simulink model "quadcopter_sim"  (R2023b)
settings: Solver=ode3  StartTime=0  StopTime=20  FixedStep=0.005  RelTol=1e-3  EnableMultiTasking=on
values from neighbouring files (symbols this model uses):
  g = 9.82    [quadcopter_par.m]
  Ic_x = inertia_matrix(m_x, p_x)    [quadcopter_par.m]
  M_RB = [ mass*eye(3) , zeros(3) ; zeros(3) , Ic_x ]    [quadcopter_par.m]
  mass = sum(m_x)    [quadcopter_par.m]
libraries: aerolibutil x14, sharedtransform x13, slpidlib x6, sharedutil x6, simulink_extras x5, matrix_library x5, vrlib x2, shareduavrstlib x1
(part 2 of 2)

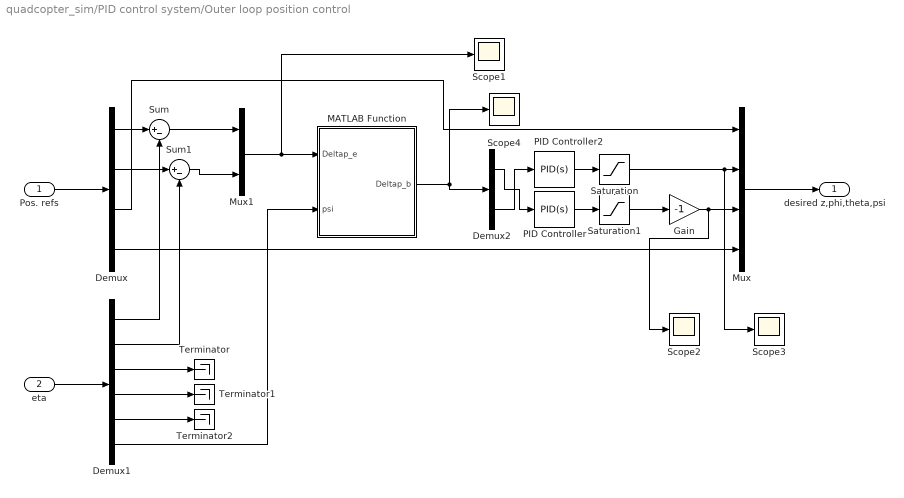
== system quadcopter_sim/PID control system/Outer loop position control ==
  Pos. refs : Inport
  eta : Inport  Port=2
  Demux : Demux
  Demux1 : Demux  Outputs=6
  Demux2 : Demux  Outputs=2
  Gain : Gain  Gain=-1
  MATLAB Function : MATLAB Function  TreatAsAtomicUnit=on
  Mux : Mux
  Mux1 : Mux  Inputs=2
  PID Controller : slpidlib/PID Controller  Controller=PID  Form=Parallel  TimeDomain=Continuous-time  UseExternalTs=off  SampleTime=-1  IntegratorMethod=Forward Euler  FilterMethod=Forward Euler  ControllerParametersSource=internal  P=10  I=0  UseKiTs=off  D=20  N=100  UseFilter=on  TunerSelectOption=Transfer Function Based (PID Tuner App)  InitialConditionSource=internal  InitialConditionForIntegrator=0  InitialConditionForFilter=0  DifferentiatorICPrevScaledInput=0  ExternalReset=none  TrackingMode=off  Kt=1  LimitOutput=off  SatLimitsSource=internal  UpperSaturationLimit=100  LowerSaturationLimit=-100  LinearizeAsGain=on  AntiWindupMode=none  Kb=1  LimitIntegrator=off  UpperIntegratorSaturationLimit=inf  LowerIntegratorSaturationLimit=-inf  POutMin=[]  POutMax=[]  IOutMin=[]  IOutMax=[]  DOutMin=[]  DOutMax=[]  NOutMin=[]  NOutMax=[]  SumOutMin=[]  SumOutMax=[]  SaturationOutMin=[]  SaturationOutMax=[]  PParamMin=[]  PParamMax=[]  IParamMin=[]  IParamMax=[]  DParamMin=[]  DParamMax=[]  NParamMin=[]  NParamMax=[]  KbParamMin=[]  KbParamMax=[]  KtParamMin=[]  KtParamMax=[]  KbOutMin=[]  KbOutMax=[]  KtOutMin=[]  KtOutMax=[]  IntegratorOutMin=[]  IntegratorOutMax=[]  FilterOutMin=[]  FilterOutMax=[]  SumI1OutMin=[]  SumI1OutMax=[]  SumI2OutMin=[]  SumI2OutMax=[]  SumI3OutMin=[]  SumI3OutMax=[]  SumI4OutMin=[]  SumI4OutMax=[]  SumDOutMin=[]  SumDOutMax=[]  DifferentiatorOutMin=[]  DifferentiatorOutMax=[]  FilterDiffOutCoefMin=[]  FilterDiffOutCoefMax=[]  ReciprocalOutMin=[]  ReciprocalOutMax=[]  SumDenOutMin=[]  SumDenOutMax=[]  SumNumOutMin=[]  SumNumOutMax=[]  DivideOutMin=[]  DivideOutMax=[]  UdiffTsProdOutMin=[]  UdiffTsProdOutMax=[]  NTsProdOutMin=[]  NTsProdOutMax=[]  UintegralTsProdOutMin=[]  UintegralTsProdOutMax=[]  UngainTsProdOutMin=[]  UngainTsProdOutMax=[]  ClampingZeroOutDataTypeStr=Inherit: Inherit via back propagation  ClampingZeroOutMin=[]  ClampingZeroOutMax=[]  FilterDenConstantOutDataTypeStr=Inherit: Inherit via back propagation  FilterDenConstantOutMin=[]  FilterDenConstantOutMax=[]  PCopyOutDataTypeStr=Inherit: Inherit via back propagation  PCopyOutMin=[]  PCopyOutMax=[]  NCopyOutDataTypeStr=Inherit: Inherit via back propagation  NCopyOutMin=[]  NCopyOutMax=[]  IntegratorContinuousStateAttributes=''  IntegratorStateMustResolveToSignalObject=off  IntegratorRTWStateStorageClass=Auto  FilterContinuousStateAttributes=''  FilterStateMustResolveToSignalObject=off  FilterRTWStateStorageClass=Auto  ParallelPVariant=InternalParameters  IdealPVariant=Disabled  IVariant=InternalParameters  DVariant=InternalParameters  IntegratorVariant=Continuous  SatVariant=Disabled  AWVariant=Passthrough  PCopyVariant=Disabled  TRVariant=Disabled  FdbkBlocksVariant=Forward  IdealPFdbkVariant=Disabled  SatFdbkVariant=Disabled  DerivativeFilterVariant=ContFilter  NVariant=InternalParameters  NCopyVariant=Disabled  FilterICVariant=InternalICsFilter  IntegratorICVariant=InternalICs  ExternalResetVariant=Disabled  TRSumVariant=Passthrough  SumFdbkVariant=Disabled  SumVariant=Sum_PID  TsampFilterVariant=InternalTs  TsampNgainVariant=Passthrough  TsampIntegralVariant=Disabled_SignalSpec  ExternalSaturationOutDataTypeStr=Inherit: Same as second input
  PID Controller2 : slpidlib/PID Controller  Controller=PID  Form=Parallel  TimeDomain=Continuous-time  UseExternalTs=off  SampleTime=-1  IntegratorMethod=Forward Euler  FilterMethod=Forward Euler  ControllerParametersSource=internal  P=10  I=0  UseKiTs=off  D=20  N=100  UseFilter=on  TunerSelectOption=Transfer Function Based (PID Tuner App)  InitialConditionSource=internal  InitialConditionForIntegrator=0  InitialConditionForFilter=0  DifferentiatorICPrevScaledInput=0  ExternalReset=none  TrackingMode=off  Kt=1  LimitOutput=off  SatLimitsSource=internal  UpperSaturationLimit=100  LowerSaturationLimit=-100  LinearizeAsGain=on  AntiWindupMode=none  Kb=1  LimitIntegrator=off  UpperIntegratorSaturationLimit=inf  LowerIntegratorSaturationLimit=-inf  POutMin=[]  POutMax=[]  IOutMin=[]  IOutMax=[]  DOutMin=[]  DOutMax=[]  NOutMin=[]  NOutMax=[]  SumOutMin=[]  SumOutMax=[]  SaturationOutMin=[]  SaturationOutMax=[]  PParamMin=[]  PParamMax=[]  IParamMin=[]  IParamMax=[]  DParamMin=[]  DParamMax=[]  NParamMin=[]  NParamMax=[]  KbParamMin=[]  KbParamMax=[]  KtParamMin=[]  KtParamMax=[]  KbOutMin=[]  KbOutMax=[]  KtOutMin=[]  KtOutMax=[]  IntegratorOutMin=[]  IntegratorOutMax=[]  FilterOutMin=[]  FilterOutMax=[]  SumI1OutMin=[]  SumI1OutMax=[]  SumI2OutMin=[]  SumI2OutMax=[]  SumI3OutMin=[]  SumI3OutMax=[]  SumI4OutMin=[]  SumI4OutMax=[]  SumDOutMin=[]  SumDOutMax=[]  DifferentiatorOutMin=[]  DifferentiatorOutMax=[]  FilterDiffOutCoefMin=[]  FilterDiffOutCoefMax=[]  ReciprocalOutMin=[]  ReciprocalOutMax=[]  SumDenOutMin=[]  SumDenOutMax=[]  SumNumOutMin=[]  SumNumOutMax=[]  DivideOutMin=[]  DivideOutMax=[]  UdiffTsProdOutMin=[]  UdiffTsProdOutMax=[]  NTsProdOutMin=[]  NTsProdOutMax=[]  UintegralTsProdOutMin=[]  UintegralTsProdOutMax=[]  UngainTsProdOutMin=[]  UngainTsProdOutMax=[]  ClampingZeroOutDataTypeStr=Inherit: Inherit via back propagation  ClampingZeroOutMin=[]  ClampingZeroOutMax=[]  FilterDenConstantOutDataTypeStr=Inherit: Inherit via back propagation  FilterDenConstantOutMin=[]  FilterDenConstantOutMax=[]  PCopyOutDataTypeStr=Inherit: Inherit via back propagation  PCopyOutMin=[]  PCopyOutMax=[]  NCopyOutDataTypeStr=Inherit: Inherit via back propagation  NCopyOutMin=[]  NCopyOutMax=[]  IntegratorContinuousStateAttributes=''  IntegratorStateMustResolveToSignalObject=off  IntegratorRTWStateStorageClass=Auto  FilterContinuousStateAttributes=''  FilterStateMustResolveToSignalObject=off  FilterRTWStateStorageClass=Auto  ParallelPVariant=InternalParameters  IdealPVariant=Disabled  IVariant=InternalParameters  DVariant=InternalParameters  IntegratorVariant=Continuous  SatVariant=Disabled  AWVariant=Passthrough  PCopyVariant=Disabled  TRVariant=Disabled  FdbkBlocksVariant=Forward  IdealPFdbkVariant=Disabled  SatFdbkVariant=Disabled  DerivativeFilterVariant=ContFilter  NVariant=InternalParameters  NCopyVariant=Disabled  FilterICVariant=InternalICsFilter  IntegratorICVariant=InternalICs  ExternalResetVariant=Disabled  TRSumVariant=Passthrough  SumFdbkVariant=Disabled  SumVariant=Sum_PID  TsampFilterVariant=InternalTs  TsampNgainVariant=Passthrough  TsampIntegralVariant=Disabled_SignalSpec  ExternalSaturationOutDataTypeStr=Inherit: Same as second input
  Saturation : Saturate  UpperLimit=10  LowerLimit=-10
  Saturation1 : Saturate  UpperLimit=10  LowerLimit=-10
  Scope{1..4} (4 alike) : Scope
  Sum : Sum  Inputs=|+-
  Sum1 : Sum  Inputs=|+-
  Terminator : Terminator
  Terminator1 : Terminator
  Terminator2 : Terminator
  desired z,phi,theta,psi : Outport
  wires:
  Demux1/3 -> Terminator/1
  Demux1/5 -> Terminator2/1
  Pos. refs/1 -> Demux/1
  Demux1/2 -> Sum1/2
  Demux1/4 -> Terminator1/1
  Demux1/1 -> Sum/2
  eta/1 -> Demux1/1
  Mux/1 -> desired z,phi,theta,psi/1
  PID Controller/1 -> Saturation1/1
  PID Controller2/1 -> Saturation/1
  Saturation1/1 -> Gain/1
  Gain/1 -> Scope2/1, Mux/3
  Demux/3 -> Mux/1
  Demux/4 -> Mux/4
  Demux/1 -> Sum/1
  Demux/2 -> Sum1/1
  Sum/1 -> Mux1/1
  Sum1/1 -> Mux1/2
  MATLAB Function/1(Deltap_b) -> Demux2/1, Scope4/1
  Mux1/1 -> Scope1/1, MATLAB Function/1(Deltap_e)
  Demux1/6 -> MATLAB Function/2(psi)
  Saturation/1 -> Scope3/1, Mux/2
  Demux2/2 -> PID Controller2/1
  Demux2/1 -> PID Controller/1

== system quadcopter_sim/Quadcopter model/Kinematics ==
  nu : Inport
  init. cond. : Inport  Port=2
  Integrator : Integrator  InitialConditionSource=external  InitialCondition=[0;0;-10;0;pi/2;0]
  Kinematics : MATLAB Function  TreatAsAtomicUnit=on
  R_be : Outport
  eta : Outport  Port=2
  wires:
  Kinematics/1(R_be) -> R_be/1
  Kinematics/2(eta_dot) -> Integrator/1
  nu/1 -> Kinematics/1(nu)
  init. cond./1 -> Integrator/2
  Integrator/1 -> eta/1, Kinematics/2(eta)

== system quadcopter_sim/Quadcopter model/Rigid-body dynamics ==
  note: $\nu$
  tau_g : Inport
  tau_p : Inport  Port=2
  Constant : Constant  Value=mass
  Constant1 : Constant  Value=Ic_x  VectorParams1D=off
  Coriolis term : MATLAB Function  TreatAsAtomicUnit=on
  Gain : Gain  Gain=inv(M_RB)  Multiplication=Matrix(K*u) (u vector)
  Integrator1 : Integrator  InitialCondition=[0;0;0;0;0;0]
  Sum : Sum  Inputs=++-
  nu : Outport
  wires:
  Integrator1/1 -> nu/1, Coriolis term/1(nu)
  Constant/1 -> Coriolis term/2(m)
  Sum/1 -> Gain/1
  tau_p/1 -> Sum/2
  Coriolis term/1(Cnunu) -> Sum/3
  Constant1/1 -> Coriolis term/3(Ic)
  Gain/1 -> Integrator1/1
  tau_g/1 -> Sum/1

== system quadcopter_sim/Quadcopter model/gravity ==
  R_be : Inport
  Manual Switch : ManualSwitch
  Math Function : Math  Operator=transpose
  Matrix Multiply : Product  Multiplication=Matrix(*)
  Mux2 : Mux  Inputs=2
  gravity vector : Constant  Value=[0;0;mass*9.82]  VectorParams1D=off
  zeros : Constant  Value=[0;0;0]  VectorParams1D=off
  tau_g : Outport
  wires:
  Matrix Multiply/1 -> Manual Switch/1
  Manual Switch/1 -> Mux2/1
  Mux2/1 -> tau_g/1
  gravity vector/1 -> Matrix Multiply/2
  zeros/1 -> Mux2/2, Manual Switch/2
  Math Function/1 -> Matrix Multiply/1
  R_be/1 -> Math Function/1

== system quadcopter_sim/Quadcopter model from paper/Kinematics working ==
  nu : Inport
  init. cond. : Inport  Port=2
  Anglesl to rot matrix : MATLAB Function  TreatAsAtomicUnit=on
  Demux1 : Demux  Outputs=2
  Integrator2 : Integrator  InitialConditionSource=external  InitialCondition=[0;0;-10;0;pi/2;0]
  Kinematics : MATLAB Function  TreatAsAtomicUnit=on
  Matrix Multiply : Product  Multiplication=Matrix(*)
  Mux : Mux  Inputs=2
  R_be : Outport
  eta : Outport  Port=2
  wires:
  Anglesl to rot matrix/1(R_be) -> Matrix Multiply/1, R_be/1
  nu/1 -> Demux1/1
  Demux1/1 -> Matrix Multiply/2
  Matrix Multiply/1 -> Mux/1
  Demux1/2 -> Kinematics/1(omega_dot)
  Kinematics/1(Theta_dot) -> Mux/2
  Mux/1 -> Integrator2/1
  init. cond./1 -> Integrator2/2
  Integrator2/1 -> Anglesl to rot matrix/1(eta), Kinematics/2(eta), eta/1

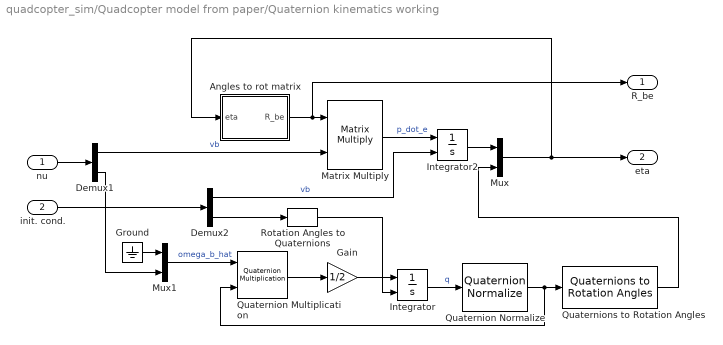
== system quadcopter_sim/Quadcopter model from paper/Quaternion kinematics working ==
  nu : Inport
  init. cond. : Inport  Port=2
  Angles to rot matrix : MATLAB Function  TreatAsAtomicUnit=on
  Demux1 : Demux  Outputs=2
  Demux2 : Demux  Outputs=2
  Gain : Gain  Gain=1/2
  Ground : Ground
  Integrator : Integrator  InitialConditionSource=external  InitialCondition=[1;0;0;0]
  Integrator2 : Integrator  InitialConditionSource=external  InitialCondition=[0;0;-10;0;pi/2;0]
  Matrix Multiply : Product  Multiplication=Matrix(*)
  Mux : Mux  Inputs=2
  Mux1 : Mux  Inputs=2
  Quaternion Multiplication : aerolibutil/Quaternion Multiplication
  Quaternion Normalize : sharedutil/Quaternion Normalize  aMode=aMode
  Quaternions to Rotation Angles : sharedtransform/Quaternions to Rotation Angles  rotationOrder=XYZ  aMode=aMode
  Rotation Angles to Quaternions : sharedtransform/Rotation Angles to Quaternions  rotationOrder=XYZ  aMode=aMode
  R_be : Outport
  eta : Outport  Port=2
  wires:
  Angles to rot matrix/1(R_be) -> Matrix Multiply/1, R_be/1
  nu/1 -> Demux1/1
  Demux1/1 -> Matrix Multiply/2  "vb"
  Ground/1 -> Mux1/1
  Demux1/2 -> Mux1/2
  Mux1/1 -> Quaternion Multiplication/1  "omega_b_hat"
  Quaternion Multiplication/1 -> Gain/1
  Gain/1 -> Integrator/1
  Integrator/1 -> Quaternion Normalize/1  "q"
  Matrix Multiply/1 -> Integrator2/1  "p_dot_e"
  Integrator2/1 -> Mux/1
  Mux/1 -> Angles to rot matrix/1(eta), eta/1
  init. cond./1 -> Demux2/1
  Demux2/1 -> Integrator2/2  "vb"
  Quaternions to Rotation Angles/1 -> Mux/2
  Quaternion Normalize/1 -> Quaternions to Rotation Angles/1, Quaternion Multiplication/2
  Demux2/2 -> Rotation Angles to Quaternions/1
  Rotation Angles to Quaternions/1 -> Integrator/2

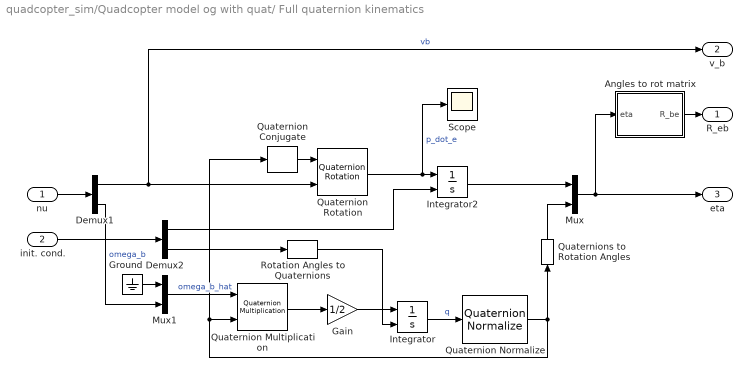
== system quadcopter_sim/Quadcopter model og with quat/ Full quaternion kinematics ==
  nu : Inport
  init. cond. : Inport  Port=2
  Angles to rot matrix : MATLAB Function  TreatAsAtomicUnit=on
  Demux1 : Demux  Outputs=2
  Demux2 : Demux  Outputs=2
  Gain : Gain  Gain=1/2
  Ground : Ground
  Integrator : Integrator  InitialConditionSource=external  InitialCondition=[1;0;0;0]
  Integrator2 : Integrator  InitialConditionSource=external  InitialCondition=[0;0;-10;0;pi/2;0]
  Mux : Mux  Inputs=2
  Mux1 : Mux  Inputs=2
  Quaternion Conjugate : aerolibutil/Quaternion Conjugate
  Quaternion Multiplication : aerolibutil/Quaternion Multiplication
  Quaternion Normalize : sharedutil/Quaternion Normalize  aMode=aMode
  Quaternion Rotation : aerolibutil/Quaternion Rotation
  Quaternions to Rotation Angles : sharedtransform/Quaternions to Rotation Angles  rotationOrder=XYZ  aMode=aMode
  Rotation Angles to Quaternions : sharedtransform/Rotation Angles to Quaternions  rotationOrder=XYZ  aMode=aMode
  Scope : Scope
  R_eb : Outport
  v_b : Outport  Port=2
  eta : Outport  Port=3
  wires:
  nu/1 -> Demux1/1
  Demux1/1 -> v_b/1, Quaternion Rotation/2  "vb"
  Ground/1 -> Mux1/1
  Demux1/2 -> Mux1/2  "omega_b"
  Mux1/1 -> Quaternion Multiplication/1  "omega_b_hat"
  Quaternion Multiplication/1 -> Gain/1
  Gain/1 -> Integrator/1
  Integrator/1 -> Quaternion Normalize/1  "q"
  Quaternion Rotation/1 -> Scope/1, Integrator2/1  "p_dot_e"
  Integrator2/1 -> Mux/1
  Mux/1 -> Angles to rot matrix/1(eta), eta/1
  init. cond./1 -> Demux2/1
  Demux2/1 -> Integrator2/2
  Quaternions to Rotation Angles/1 -> Mux/2
  Quaternion Normalize/1 -> Quaternion Conjugate/1, Quaternion Multiplication/2, Quaternions to Rotation Angles/1
  Demux2/2 -> Rotation Angles to Quaternions/1
  Rotation Angles to Quaternions/1 -> Integrator/2
  Angles to rot matrix/1(R_be) -> R_eb/1
  Quaternion Conjugate/1 -> Quaternion Rotation/1

== system quadcopter_sim/Quadcopter model og with quat/Kinematics working ==
  nu : Inport
  init. cond. : Inport  Port=2
  Anglesl to rot matrix : MATLAB Function  TreatAsAtomicUnit=on
  Demux1 : Demux  Outputs=2
  Integrator2 : Integrator  InitialConditionSource=external  InitialCondition=[0;0;-10;0;pi/2;0]
  Kinematics : MATLAB Function  TreatAsAtomicUnit=on
  Matrix Multiply : Product  Multiplication=Matrix(*)
  Mux : Mux  Inputs=2
  R_be : Outport
  eta : Outport  Port=2
  wires:
  Anglesl to rot matrix/1(R_be) -> Matrix Multiply/1, R_be/1
  nu/1 -> Demux1/1
  Demux1/1 -> Matrix Multiply/2
  Matrix Multiply/1 -> Mux/1
  Demux1/2 -> Kinematics/1(omega_dot)
  Kinematics/1(Theta_dot) -> Mux/2
  Mux/1 -> Integrator2/1
  init. cond./1 -> Integrator2/2
  Integrator2/1 -> Anglesl to rot matrix/1(eta), Kinematics/2(eta), eta/1

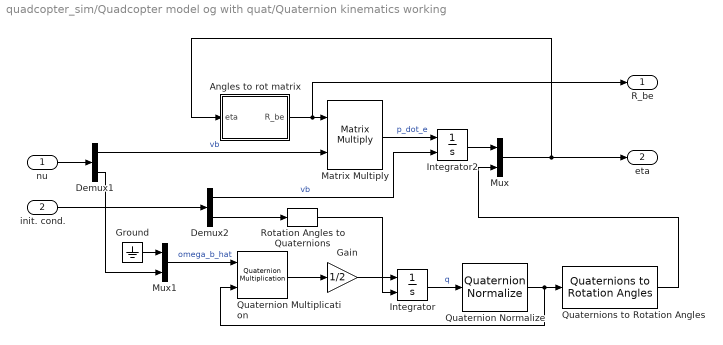
== system quadcopter_sim/Quadcopter model og with quat/Quaternion kinematics working ==
  nu : Inport
  init. cond. : Inport  Port=2
  Angles to rot matrix : MATLAB Function  TreatAsAtomicUnit=on
  Demux1 : Demux  Outputs=2
  Demux2 : Demux  Outputs=2
  Gain : Gain  Gain=1/2
  Ground : Ground
  Integrator : Integrator  InitialConditionSource=external  InitialCondition=[1;0;0;0]
  Integrator2 : Integrator  InitialConditionSource=external  InitialCondition=[0;0;-10;0;pi/2;0]
  Matrix Multiply : Product  Multiplication=Matrix(*)
  Mux : Mux  Inputs=2
  Mux1 : Mux  Inputs=2
  Quaternion Multiplication : aerolibutil/Quaternion Multiplication
  Quaternion Normalize : sharedutil/Quaternion Normalize  aMode=aMode
  Quaternions to Rotation Angles : sharedtransform/Quaternions to Rotation Angles  rotationOrder=XYZ  aMode=aMode
  Rotation Angles to Quaternions : sharedtransform/Rotation Angles to Quaternions  rotationOrder=XYZ  aMode=aMode
  R_be : Outport
  eta : Outport  Port=2
  wires:
  Angles to rot matrix/1(R_be) -> Matrix Multiply/1, R_be/1
  nu/1 -> Demux1/1
  Demux1/1 -> Matrix Multiply/2  "vb"
  Ground/1 -> Mux1/1
  Demux1/2 -> Mux1/2
  Mux1/1 -> Quaternion Multiplication/1  "omega_b_hat"
  Quaternion Multiplication/1 -> Gain/1
  Gain/1 -> Integrator/1
  Integrator/1 -> Quaternion Normalize/1  "q"
  Matrix Multiply/1 -> Integrator2/1  "p_dot_e"
  Integrator2/1 -> Mux/1
  Mux/1 -> Angles to rot matrix/1(eta), eta/1
  init. cond./1 -> Demux2/1
  Demux2/1 -> Integrator2/2  "vb"
  Quaternions to Rotation Angles/1 -> Mux/2
  Quaternion Normalize/1 -> Quaternions to Rotation Angles/1, Quaternion Multiplication/2
  Demux2/2 -> Rotation Angles to Quaternions/1
  Rotation Angles to Quaternions/1 -> Integrator/2

== system quadcopter_sim/Quadcopter model og with quat/Rigid-body dynamics ==
  note: $\nu$
  tau_g : Inport
  tau_d : Inport  Port=2
  tau_p : Inport  Port=3
  Constant : Constant  Value=mass
  Constant1 : Constant  Value=Ic_x  VectorParams1D=off
  Coriolis term : MATLAB Function  TreatAsAtomicUnit=on
  Gain : Gain  Gain=inv(M_RB)  Multiplication=Matrix(K*u) (u vector)
  Integrator1 : Integrator  InitialCondition=[0;0;0.001;0;0;0]
  Sum : Sum  Inputs=++-
  Sum1 : Sum  Inputs=++|
  nu : Outport
  wires:
  Integrator1/1 -> nu/1, Coriolis term/1(nu)
  Constant/1 -> Coriolis term/2(m)
  Sum/1 -> Gain/1
  Coriolis term/1(Cnunu) -> Sum/3
  Constant1/1 -> Coriolis term/3(Ic)
  Gain/1 -> Integrator1/1
  tau_g/1 -> Sum/1
  Sum1/1 -> Sum/2
  tau_p/1 -> Sum1/2
  tau_d/1 -> Sum1/1

== system quadcopter_sim/Quadcopter model og with quat/drag ==
  v_b : Inport
  Air density : Gain  Gain=1.204
  Divide : Product  Inputs=*/
  Dot Product : DotProduct  OutDataTypeStr=Inherit: Inherit via internal rule
  Drag coeffecient * area : Gain  Gain=5
  Gain : Gain  Gain=1/2
  Manual Switch : ManualSwitch  CurrentSetting=0
  Mux2 : Mux  Inputs=2
  Product : Product
  Reverse : Gain  Gain=-1
  Scope : Scope
  Scope1 : Scope
  Sqrt : Sqrt
  zeros : Constant  Value=[0;0;0]  VectorParams1D=off
  tau_d : Outport
  wires:
  Manual Switch/1 -> Mux2/1
  Mux2/1 -> tau_d/1
  zeros/1 -> Mux2/2, Manual Switch/2
  v_b/1 -> Divide/1, Dot Product/1, Dot Product/2
  Dot Product/1 -> Gain/1, Sqrt/1
  Gain/1 -> Air density/1
  Air density/1 -> Drag coeffecient * area/1
  Product/1 -> Scope/1, Manual Switch/1
  Drag coeffecient * area/1 -> Product/1, Scope1/1
  Sqrt/1 -> Divide/2
  Divide/1 -> Reverse/1
  Reverse/1 -> Product/2

== system quadcopter_sim/Quadcopter model og with quat/gravity ==
  R_eb : Inport
  Manual Switch : ManualSwitch
  Math Function : Math  Operator=transpose
  Matrix Multiply : Product  Multiplication=Matrix(*)
  Mux2 : Mux  Inputs=2
  gravity vector : Constant  Value=[0;0;mass*9.82]  VectorParams1D=off
  zeros : Constant  Value=[0;0;0]  VectorParams1D=off
  tau_g : Outport
  wires:
  Matrix Multiply/1 -> Manual Switch/1
  Manual Switch/1 -> Mux2/1
  Mux2/1 -> tau_g/1
  gravity vector/1 -> Matrix Multiply/2
  zeros/1 -> Mux2/2, Manual Switch/2
  Math Function/1 -> Matrix Multiply/1
  R_eb/1 -> Math Function/1

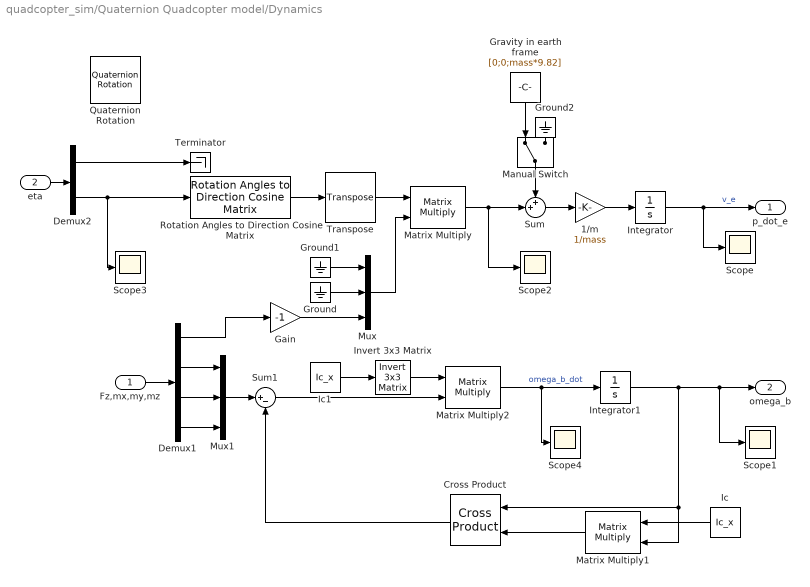
== system quadcopter_sim/Quaternion Quadcopter model/Dynamics ==
  Fz,mx,my,mz : Inport
  eta : Inport  Port=2
  1/m : Gain  Gain=1/mass
  Cross Product : matrix_library/Cross Product
  Demux1 : Demux
  Demux2 : Demux  Outputs=2
  Gain : Gain  Gain=-1
  Gravity in earth frame : Constant  Value=[0;0;mass*9.82]
  Ground : Ground
  Ground1 : Ground
  Ground2 : Ground
  Ic : Constant  Value=Ic_x
  Ic1 : Constant  Value=Ic_x
  Integrator : Integrator  InitialCondition=[0;0;0]
  Integrator1 : Integrator  InitialCondition=[0;0;0]
  Invert 3x3 Matrix : aerolibutil/Invert  3x3 Matrix
  Manual Switch : ManualSwitch
  Matrix Multiply : Product  Multiplication=Matrix(*)
  Matrix Multiply1 : Product  Multiplication=Matrix(*)
  Matrix Multiply2 : Product  Multiplication=Matrix(*)
  Mux : Mux  Inputs=3
  Mux1 : Mux  Inputs=3
  Quaternion Rotation : aerolibutil/Quaternion Rotation
  Rotation Angles to Direction Cosine Matrix : sharedtransform/Rotation Angles to Direction Cosine Matrix  rotationOrder=XYZ  aMode=aMode
  Scope{,1..4} (5 alike) : Scope
  Sum : Sum  Inputs=++|
  Sum1 : Sum  Inputs=|+-
  Terminator : Terminator
  Transpose : matrix_library/Transpose
  p_dot_e : Outport
  omega_b : Outport  Port=2
  wires:
  Demux1/1 -> Gain/1
  Gain/1 -> Mux/3
  Ground/1 -> Mux/2
  Ground1/1 -> Mux/1
  Manual Switch/1 -> Sum/1
  Sum/1 -> 1/m/1
  Integrator/1 -> Scope/1, p_dot_e/1  "v_e"
  Integrator1/1 -> Matrix Multiply1/2, Cross Product/1, Scope1/1, omega_b/1
  Mux1/1 -> Sum1/1
  Ic/1 -> Matrix Multiply1/1
  Matrix Multiply1/1 -> Cross Product/2
  Cross Product/1 -> Sum1/2
  Sum1/1 -> Matrix Multiply2/2
  Invert 3x3 Matrix/1 -> Matrix Multiply2/1
  Ic1/1 -> Invert 3x3 Matrix/1
  Matrix Multiply2/1 -> Scope4/1, Integrator1/1  "omega_b_dot"
  Gravity in earth frame/1 -> Manual Switch/1
  1/m/1 -> Integrator/1
  Fz,mx,my,mz/1 -> Demux1/1
  Demux1/2 -> Mux1/1
  Demux1/3 -> Mux1/2
  Demux1/4 -> Mux1/3
  Mux/1 -> Matrix Multiply/2
  eta/1 -> Demux2/1
  Matrix Multiply/1 -> Scope2/1, Sum/2
  Demux2/1 -> Terminator/1
  Demux2/2 -> Scope3/1, Rotation Angles to Direction Cosine Matrix/1
  Rotation Angles to Direction Cosine Matrix/1 -> Transpose/1
  Transpose/1 -> Matrix Multiply/1

== system quadcopter_sim/Quaternion Quadcopter model/Quaternion-based Kinematics ==
  p_dot_e : Inport
  omega_b : Inport  Port=2
  p0_e : Inport  Port=3
  r0_e : Inport  Port=4
  Gain : Gain  Gain=1/2
  Ground : Ground
  Integrator : Integrator  InitialConditionSource=external
  Integrator1 : Integrator  InitialConditionSource=external
  Mux : Mux  Inputs=2
  Mux1 : Mux  Inputs=2
  Quaternion Multiplication : aerolibutil/Quaternion Multiplication
  Quaternion Normalize : sharedutil/Quaternion Normalize  aMode=aMode
  Quaternions to Rotation Angles : sharedtransform/Quaternions to Rotation Angles  rotationOrder=XYZ  aMode=aMode
  Rotation Angles to Quaternions : sharedtransform/Rotation Angles to Quaternions  rotationOrder=XYZ  aMode=aMode
  Scope : Scope
  eta : Outport
  q : Outport  Port=2
  wires:
  omega_b/1 -> Mux/2
  Ground/1 -> Mux/1
  p_dot_e/1 -> Integrator/1
  p0_e/1 -> Integrator/2
  Integrator1/1 -> Quaternion Normalize/1  "q"
  Quaternion Multiplication/1 -> Gain/1
  Gain/1 -> Integrator1/1
  r0_e/1 -> Rotation Angles to Quaternions/1
  Rotation Angles to Quaternions/1 -> Integrator1/2
  Mux1/1 -> eta/1
  Integrator/1 -> Mux1/1  "p_e"
  Quaternions to Rotation Angles/1 -> Scope/1, Mux1/2  "Theta_e"
  Quaternion Normalize/1 -> Quaternion Multiplication/2, q/1, Quaternions to Rotation Angles/1
  Mux/1 -> Quaternion Multiplication/1  "omega_b_hat"

== system quadcopter_sim/Quaternion2/Dynamics ==
  Fz,mx,my,mz : Inport
  q : Inport  Port=2
  Cross Product : matrix_library/Cross Product
  Demux1 : Demux
  Gain : Gain  Gain=[0;0;1/mass]
  Gravity : Constant  Value=[0; 0; -9.82]
  Ic_x : Gain  Gain=Ic_x  Multiplication=Matrix(K*u)
  Integrator : Integrator
  Integrator1 : Integrator
  Mux1 : Mux  Inputs=3
  Quaternion Rotation : aerolibutil/Quaternion Rotation
  Scope : Scope
  Sum : Sum  Inputs=|+-
  Sum1 : Sum  Inputs=++|
  inv(Ic_x) : Gain  Gain=inv(Ic_x)  Multiplication=Matrix(K*u) (u vector)
  p_dot_e : Outport
  omega_b : Outport  Port=2
  wires:
  Fz,mx,my,mz/1 -> Demux1/1
  Demux1/2 -> Mux1/1
  Demux1/3 -> Mux1/2
  Demux1/4 -> Mux1/3
  Integrator1/1 -> Cross Product/1, Scope/1, Ic_x/1, omega_b/1
  Mux1/1 -> Sum/1
  Ic_x/1 -> Cross Product/2
  Cross Product/1 -> Sum/2
  Sum/1 -> inv(Ic_x)/1
  inv(Ic_x)/1 -> Integrator1/1
  Gravity/1 -> Sum1/1
  Demux1/1 -> Gain/1
  Quaternion Rotation/1 -> Sum1/2
  Integrator/1 -> p_dot_e/1
  Sum1/1 -> Integrator/1
  q/1 -> Quaternion Rotation/1
  Gain/1 -> Quaternion Rotation/2

== system quadcopter_sim/Quaternion2/Quaternion-based Kinematics ==
  p_dot_e : Inport
  omega_b : Inport  Port=2
  p0_e : Inport  Port=3
  r0_e : Inport  Port=4
  Gain : Gain  Gain=1/2
  Ground : Ground
  Integrator : Integrator  InitialConditionSource=external
  Integrator1 : Integrator  InitialConditionSource=external
  Mux : Mux  Inputs=2
  Mux1 : Mux  Inputs=2
  Quaternion Multiplication : aerolibutil/Quaternion Multiplication
  Quaternion Normalize : sharedutil/Quaternion Normalize  aMode=aMode
  Quaternions to Rotation Angles : sharedtransform/Quaternions to Rotation Angles  rotationOrder=XYZ  aMode=aMode
  Rotation Angles to Quaternions : sharedtransform/Rotation Angles to Quaternions  rotationOrder=XYZ  aMode=aMode
  Scope : Scope
  eta : Outport
  q : Outport  Port=2
  wires:
  omega_b/1 -> Mux/2
  Ground/1 -> Mux/1
  p_dot_e/1 -> Integrator/1
  p0_e/1 -> Integrator/2
  Integrator1/1 -> Quaternion Normalize/1  "q"
  Quaternion Multiplication/1 -> Gain/1
  Gain/1 -> Integrator1/1
  r0_e/1 -> Rotation Angles to Quaternions/1
  Rotation Angles to Quaternions/1 -> Integrator1/2
  Mux1/1 -> eta/1
  Integrator/1 -> Mux1/1  "p_e"
  Quaternions to Rotation Angles/1 -> Scope/1, Mux1/2  "Theta_e"
  Quaternion Normalize/1 -> q/1, Quaternion Multiplication/2, Quaternions to Rotation Angles/1
  Mux/1 -> Quaternion Multiplication/1  "omega_b_hat"

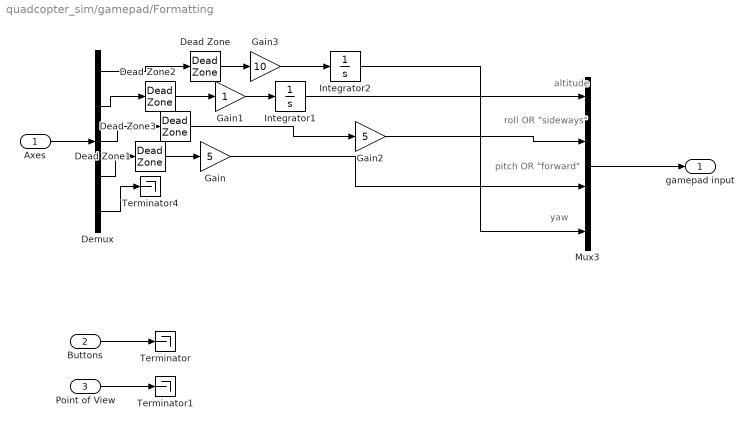
== system quadcopter_sim/gamepad/Formatting ==
  note: roll OR "sideways"
  note: altitude
  note: pitch OR "forward"
  note: yaw
  Axes : Inport
  Buttons : Inport  Port=2
  Point of View : Inport  Port=3
  Dead Zone{,1..3} (4 alike) : DeadZone  LowerValue=-0.2  UpperValue=0.2
  Demux : Demux  Outputs=5
  Gain : Gain  Gain=5
  Gain1 : Gain
  Gain2 : Gain  Gain=5
  Gain3 : Gain  Gain=10
  Integrator1 : Integrator  InitialCondition=-10
  Integrator2 : Integrator
  Mux3 : Mux
  Terminator : Terminator
  Terminator1 : Terminator
  Terminator4 : Terminator
  gamepad input : Outport
  wires:
  Mux3/1 -> gamepad input/1
  Buttons/1 -> Terminator/1
  Axes/1 -> Demux/1
  Demux/3 -> Dead Zone3/1
  Demux/5 -> Terminator4/1
  Demux/4 -> Dead Zone1/1
  Demux/1 -> Dead Zone/1
  Dead Zone1/1 -> Gain/1
  Demux/2 -> Dead Zone2/1
  Dead Zone2/1 -> Gain1/1
  Integrator1/1 -> Mux3/1
  Dead Zone/1 -> Gain3/1
  Integrator2/1 -> Mux3/4
  Dead Zone3/1 -> Gain2/1
  Point of View/1 -> Terminator1/1
  Gain1/1 -> Integrator1/1
  Gain2/1 -> Mux3/2
  Gain/1 -> Mux3/3
  Gain3/1 -> Integrator2/1

== system quadcopter_sim/Formatting/Euler to VR/Axis Angle Vector ==
  e0 : Inport
  2 : Gain  Gain=2  SaturateOnIntegerOverflow=on  OutDataTypeStr=Inherit: Same as input  ParamDataTypeStr=Inherit: Same as input
  Constant : Constant  Value=1e-6
  Demux : Demux  Outputs=[1 3 ]
      settings: DisplayOption=none
  Mux : Mux  Inputs=2
  Product : Product  Inputs=*/  InputSameDT=on  SaturateOnIntegerOverflow=on  OutDataTypeStr=Inherit: Same as first input
  Switch : Switch  Criteria=u2 ~= 0  SaturateOnIntegerOverflow=off  InputSameDT=off
  Trigonometric Function : Trigonometry
  Trigonometric Function2 : Trigonometry  Operator=acos
  e0_norm : Outport  VectorParamsAs1DForOutWhenUnconnected=off
  wires:
  Demux/1 -> Trigonometric Function2/1
  Demux/2 -> Product/1
  Mux/1 -> e0_norm/1
  Product/1 -> Mux/1
  2/1 -> Mux/2
  Trigonometric Function/1 -> Switch/1, Switch/2
  Trigonometric Function2/1 -> Trigonometric Function/1, 2/1
  e0/1 -> Demux/1
  Constant/1 -> Switch/3
  Switch/1 -> Product/2

== system quadcopter_sim/Formatting/Euler to VR/Quaternion Normalization ==
  e0 : Inport
  1/2 : Gain  Gain=1/2  SaturateOnIntegerOverflow=on  OutDataTypeStr=Inherit: Same as input  ParamDataTypeStr=Inherit: Same as input
  Demux : Demux  Outputs=[1 3]
      settings: DisplayOption=none
  Mux : Mux  Inputs=2
  Product : Product  InputSameDT=on  SaturateOnIntegerOverflow=on  OutDataTypeStr=Inherit: Same as first input
  Trigonometric Function : Trigonometry
  Trigonometric Function1 : Trigonometry  Operator=cos
  e0_norm : Outport  VectorParamsAs1DForOutWhenUnconnected=off
  wires:
  Trigonometric Function1/1 -> Mux/1
  Demux/2 -> Product/2
  Demux/1 -> 1/2/1
  Mux/1 -> e0_norm/1
  Product/1 -> Mux/2
  Trigonometric Function/1 -> Product/1
  1/2/1 -> Trigonometric Function1/1, Trigonometric Function/1
  e0/1 -> Demux/1

== system quadcopter_sim/Formatting/Euler to VR/Quaternion Normalization1 ==
  e0 : Inport
  1/2 : Gain  Gain=1/2  SaturateOnIntegerOverflow=on  OutDataTypeStr=Inherit: Same as input  ParamDataTypeStr=Inherit: Same as input
  Demux : Demux  Outputs=[1 3]
      settings: DisplayOption=none
  Mux : Mux  Inputs=2
  Product : Product  InputSameDT=on  SaturateOnIntegerOverflow=on  OutDataTypeStr=Inherit: Same as first input
  Trigonometric Function : Trigonometry
  Trigonometric Function1 : Trigonometry  Operator=cos
  e0_norm : Outport  VectorParamsAs1DForOutWhenUnconnected=off
  wires:
  e0/1 -> Demux/1
  1/2/1 -> Trigonometric Function/1, Trigonometric Function1/1
  Trigonometric Function/1 -> Product/1
  Product/1 -> Mux/2
  Mux/1 -> e0_norm/1
  Demux/1 -> 1/2/1
  Demux/2 -> Product/2
  Trigonometric Function1/1 -> Mux/1

== system quadcopter_sim/Formatting/Euler to VR/Quaternion Normalization2 ==
  e0 : Inport
  1/2 : Gain  Gain=1/2  SaturateOnIntegerOverflow=on  OutDataTypeStr=Inherit: Same as input  ParamDataTypeStr=Inherit: Same as input
  Demux : Demux  Outputs=[1 3]
      settings: DisplayOption=none
  Mux : Mux  Inputs=2
  Product : Product  InputSameDT=on  SaturateOnIntegerOverflow=on  OutDataTypeStr=Inherit: Same as first input
  Trigonometric Function : Trigonometry
  Trigonometric Function1 : Trigonometry  Operator=cos
  e0_norm : Outport  VectorParamsAs1DForOutWhenUnconnected=off
  wires:
  Trigonometric Function1/1 -> Mux/1
  Demux/2 -> Product/2
  Demux/1 -> 1/2/1
  Mux/1 -> e0_norm/1
  Product/1 -> Mux/2
  Trigonometric Function/1 -> Product/1
  1/2/1 -> Trigonometric Function1/1, Trigonometric Function/1
  e0/1 -> Demux/1

== system quadcopter_sim/PID control system/Inner-loop PID controllers/wrap_error ==
  In1 : Inport
  Trigonometric Function : Trigonometry
  Trigonometric Function1 : Trigonometry  Operator=cos
  Trigonometric Function2 : Trigonometry  Operator=atan2
  Out1 : Outport
  wires:
  In1/1 -> Trigonometric Function1/1, Trigonometric Function/1
  Trigonometric Function/1 -> Trigonometric Function2/1
  Trigonometric Function1/1 -> Trigonometric Function2/2
  Trigonometric Function2/1 -> Out1/1

== matlab function quadcopter_sim/Quadcopter model from paper/MATLAB Function ==
  data: R input; R_dot output; omega input
function R_dot = fcn(R, omega)

omega_hat = [0 -omega(3) omega(2);
             omega(3) 0 -omega(1);
             -omega(2) omega(1) 0];

R_dot = R * omega_hat;

== matlab function quadcopter_sim/Quadcopter model from paper/Kinematics working/Anglesl to rot matrix ==
  data: R_be output; eta input
function R_be = J_Theta(eta)

% Euler angle extraction
phi = eta(4);
theta = eta(5);
psi = eta(6);

R_xphi = [ 1 0 0 ; 0 cos(phi) -sin(phi) ; 0 sin(phi) cos(phi) ];
R_ytheta = [ cos(theta) 0 sin(theta) ; 0 1 0 ; -sin(theta) 0 cos(theta) ];
R_zpsi = [ cos(psi) -sin(psi) 0 ; sin(psi) cos(psi) 0 ; 0 0 1 ];

% rotation matrix
R_be = R_zpsi * R_ytheta * R_xphi;

== matlab function quadcopter_sim/Quadcopter model from paper/Kinematics working/Kinematics ==
  data: Theta_dot output; omega_dot input; eta input
function Theta_dot = J_Theta(omega_dot,eta)

% Euler angle extraction
phi = eta(4);
theta = eta(5);

% angular velocity transformation
T_Theta = [ 1 sin(phi)*tan(theta) cos(phi)*tan(theta) ; 0 cos(phi) -sin(phi) ; 0 sin(phi)/cos(theta) cos(phi)/cos(theta) ];


Theta_dot = T_Theta*omega_dot;

== matlab function quadcopter_sim/Quadcopter model from paper/Quaternion kinematics working/Angles to rot matrix ==
  data: R_be output; eta input
function R_be = J_Theta(eta)

% Euler angle extraction
phi = eta(4);
theta = eta(5);
psi = eta(6);

R_xphi = [ 1 0 0 ; 0 cos(phi) -sin(phi) ; 0 sin(phi) cos(phi) ];
R_ytheta = [ cos(theta) 0 sin(theta) ; 0 1 0 ; -sin(theta) 0 cos(theta) ];
R_zpsi = [ cos(psi) -sin(psi) 0 ; sin(psi) cos(psi) 0 ; 0 0 1 ];

% rotation matrix
R_be = R_zpsi * R_ytheta * R_xphi;

== matlab function quadcopter_sim/Quadcopter model from paper/MATLAB Function1 ==
  data: R input; z_B output
function z_B = get_z_B(R)

z_B = R(:,3);

== matlab function quadcopter_sim/Quadcopter model from paper/MATLAB Function2 ==
  data: R input; eul output
function eul = rot_to_eul(R)

eul = rotm2eul(R, 'XYZ')';

== matlab function quadcopter_sim/PID control system/Outer loop position control/MATLAB Function ==
  data: Deltap_e input; Deltap_b output; psi input
function Deltap_b = fcn(Deltap_e,psi)

R = [ cos(psi) , -sin(psi) ;
      sin(psi) ,  cos(psi) ];

Deltap_b = R'*Deltap_e;

== matlab function quadcopter_sim/Quadcopter model/Rigid-body dynamics/Coriolis term ==
  data: nu input; Cnunu output; m input; Ic input
function Cnunu = fcn(nu,m,Ic)

v = nu(1:3);  % linear velocities (expressed in the body frame)
omega = nu(4:6); % angular velocities (expressed in the body frame)


Cnunu = [ cross(omega,m*v) ; -cross(Ic*omega,omega) ];

== matlab function quadcopter_sim/Quadcopter model og with quat/ Full quaternion kinematics/Angles to rot matrix ==
  data: R_be output; eta input
function R_be = fcn(eta)

% Euler angle extraction
phi = eta(4);
theta = eta(5);
psi = eta(6);

R_xphi = [ 1 0 0 ; 0 cos(phi) -sin(phi) ; 0 sin(phi) cos(phi) ];
R_ytheta = [ cos(theta) 0 sin(theta) ; 0 1 0 ; -sin(theta) 0 cos(theta) ];
R_zpsi = [ cos(psi) -sin(psi) 0 ; sin(psi) cos(psi) 0 ; 0 0 1 ];

% rotation matrix
R_be = R_zpsi * R_ytheta * R_xphi;

== matlab function quadcopter_sim/Quadcopter model/Kinematics/Kinematics ==
  data: R_be output; nu input; eta input; eta_dot output
function [R_be,eta_dot] = J_Theta(nu,eta)

% Euler angle extraction
phi = eta(4);
theta = eta(5);
psi = eta(6);

R_xphi = [ 1 0 0 ; 0 cos(phi) -sin(phi) ; 0 sin(phi) cos(phi) ];
R_ytheta = [ cos(theta) 0 sin(theta) ; 0 1 0 ; -sin(theta) 0 cos(theta) ];
R_zpsi = [ cos(psi) -sin(psi) 0 ; sin(psi) cos(psi) 0 ; 0 0 1 ];

% rotation matrix
R_be = R_zpsi * R_ytheta * R_xphi;

% angular velocity transformation
T_Theta = [ 1 sin(phi)*tan(theta) cos(phi)*tan(theta) ; 0 cos(phi) -sin(phi) ; 0 sin(phi)/cos(theta) cos(phi)/cos(theta) ];

J_Theta = [ R_be , zeros(3) ; zeros(3) , T_Theta ];

eta_dot = J_Theta*nu;

== matlab function quadcopter_sim/Quadcopter model og with quat/Rigid-body dynamics/Coriolis term ==
  data: nu input; Cnunu output; m input; Ic input
function Cnunu = fcn(nu,m,Ic)

v = nu(1:3);  % linear velocities (expressed in the body frame)
omega = nu(4:6); % angular velocities (expressed in the body frame)


Cnunu = [ cross(omega,m*v) ; -cross(Ic*omega,omega) ];

== matlab function quadcopter_sim/Quadcopter model og with quat/Kinematics working/Anglesl to rot matrix ==
  data: R_be output; eta input
function R_be = J_Theta(eta)

% Euler angle extraction
phi = eta(4);
theta = eta(5);
psi = eta(6);

R_xphi = [ 1 0 0 ; 0 cos(phi) -sin(phi) ; 0 sin(phi) cos(phi) ];
R_ytheta = [ cos(theta) 0 sin(theta) ; 0 1 0 ; -sin(theta) 0 cos(theta) ];
R_zpsi = [ cos(psi) -sin(psi) 0 ; sin(psi) cos(psi) 0 ; 0 0 1 ];

% rotation matrix
R_be = R_zpsi * R_ytheta * R_xphi;

== matlab function quadcopter_sim/Quadcopter model og with quat/Kinematics working/Kinematics ==
  data: Theta_dot output; omega_dot input; eta input
function Theta_dot = J_Theta(omega_dot,eta)

% Euler angle extraction
phi = eta(4);
theta = eta(5);

% angular velocity transformation
T_Theta = [ 1 sin(phi)*tan(theta) cos(phi)*tan(theta) ; 0 cos(phi) -sin(phi) ; 0 sin(phi)/cos(theta) cos(phi)/cos(theta) ];


Theta_dot = T_Theta*omega_dot;

== matlab function quadcopter_sim/Quadcopter model og with quat/Quaternion kinematics working/Angles to rot matrix ==
  data: R_be output; eta input
function R_be = J_Theta(eta)

% Euler angle extraction
phi = eta(4);
theta = eta(5);
psi = eta(6);

R_xphi = [ 1 0 0 ; 0 cos(phi) -sin(phi) ; 0 sin(phi) cos(phi) ];
R_ytheta = [ cos(theta) 0 sin(theta) ; 0 1 0 ; -sin(theta) 0 cos(theta) ];
R_zpsi = [ cos(psi) -sin(psi) 0 ; sin(psi) cos(psi) 0 ; 0 0 1 ];

% rotation matrix
R_be = R_zpsi * R_ytheta * R_xphi;

== matlab function quadcopter_sim/Flat feedforward trajectory/Feedforward control signal ==
  data: p_traj input; c output; v_traj input; a_traj input; j_traj input; s_traj input; Ic input; tau output
function [c, tau]  = fcn(p_traj, v_traj, a_traj, j_traj, s_traj, Ic)

g  = 9.82;
z_W = [0; 0; 1];

psi = p_traj(4);
psi_dot = v_traj(4);
psi_ddot = a_traj(4);

p_traj = p_traj(1:3);
v_traj = v_traj(1:3);
a_traj = a_traj(1:3);
j_traj = j_traj(1:3);
s_traj = s_traj(1:3);


% Enforce heading by constraining x_B to the x_W - y_W plane.
x_C = [cos(psi); sin(psi); 0];
y_C = [-sin(psi); cos(psi); 0];

% Construct rotation matrix
alpha = a_traj + g*z_W;
beta = a_traj + g*z_W;

x_B = cross(y_C, alpha) / norm(cross(y_C, alpha));
y_B = cross(beta, x_B) / norm(cross(beta, x_B));
z_B = cross(x_B, y_B); 
R = [x_B, y_B, z_B];

% Thrust
c = z_B'*(a_traj + g*z_W);

% Angular rates
x_B_tilde = cross(y_C, z_B);

omega_x = (-1/c)*y_B'*j_traj;
omega_y = (1/c)*x_B'*j_traj;
omega_z = (1/norm(x_B_tilde))*(psi_dot*x_C'*x_B + omega_y*y_C'*z_B);
omega = [omega_x; omega_y; omega_z];

% Angular accelerations
c_dot = z_B'*j_traj;

omega_x_dot = (1/c)*(-y_B'*s_traj - 2*c_dot*omega_x + c*omega_y*omega_z);
omega_y_dot = (1/c)*(x_B'*s_traj - 2*c_dot*omega_y - c*omega_x*omega_z);
omega_z_dot = (1/norm(x_B_tilde))*(omega_y_dot*y_C'*z_B + psi_ddot*x_C'*x_B + 2*psi_dot*omega_z*x_C'*y_B - 2*psi_dot*omega_y*x_C'*z_B - omega_x*omega_y*y_C'*y_B - omega_x*omega_z*y_C'*z_B);
omega_dot = [omega_x_dot; omega_y_dot; omega_z_dot];
omega_dot = [-omega_x_dot; -omega_y_dot; omega_z_dot];

% Moments
tau = Ic*omega_dot + cross(omega, Ic*omega_dot);
